simulink model "clik_inverse"  (R2024b)
settings: Solver=ode1  StartTime=0.0  StopTime=4  FixedStep=0.001  RelTol=1e-3
undefined symbols (not defined in the file or in its folder): DiscIntNeverNeededParam, q0, Tc
settings Model: Creator=Xp  LastModifiedBy=22guo
settings SolverCC: AlgebraicLoopSolver=TrustRegion
settings DataIOCC: LimitDataPoints=on  SaveFormat=Array  SignalLoggingSaveFormat=ModelDataLogs  ReturnWorkspaceOutputs=off
settings OptimizationCC: ExpressionDepthLimit=2147483647  InitFltsAndDblsToZero=on  LifeSpan=inf
settings DebuggingCC: SaveWithParameterizedLinksMsg=none  UnderspecifiedInitializationDetection=Classic  MergeDetectMultiDrivingBlocksExec=none  SolverPrmCheckMsg=warning  MultiTaskDSMMsg=warning  MultiTaskCondExecSysMsg=none  FcnCallInpInsideContextMsg=warning  UnconnectedInputMsg=warning  UnconnectedOutputMsg=warning  UnconnectedLineMsg=warning  StateNameClashWarn=warning  SFUnexpectedBacktrackingDiag=warning  SFNoUnconditionalDefaultTransitionDiag=warning  SFExecutionAtInitializationDiag=none  ArithmeticOperatorsInVariantConditions=warning
settings HardwareCC: ProdBitPerPointer=32  ProdBitPerSizeT=32  ProdBitPerPtrDiffT=32  ProdLargestAtomicFloat=None  ProdIntDivRoundTo=Undefined  ProdEndianess=Unspecified  ProdWordSize=32  ProdHWDeviceType=32-bit Generic
settings ModelReferenceCC: EnableRefExpFcnMdlSchedulingChecks=on  PropagateSignalLabelsOutOfModel=off
settings SFSimCC: CustomCodeUndefinedFunction=UseInterfaceOnly
settings RTWCC: GPUComputeCapability=3.5  DLArmComputeVersion=19.05
settings CodeAppCC: StateflowObjectComments=on
settings GRTTargetCC: TargetLangStandard=C89/C90 (ANSI)  CombineOutputUpdateFcns=off  GRTInterface=on
settings ConfigComp: CovMetricSettings=dw  CovSaveCumulativeToWorkspaceVar=on  CovSaveSingleToWorkspaceVar=on

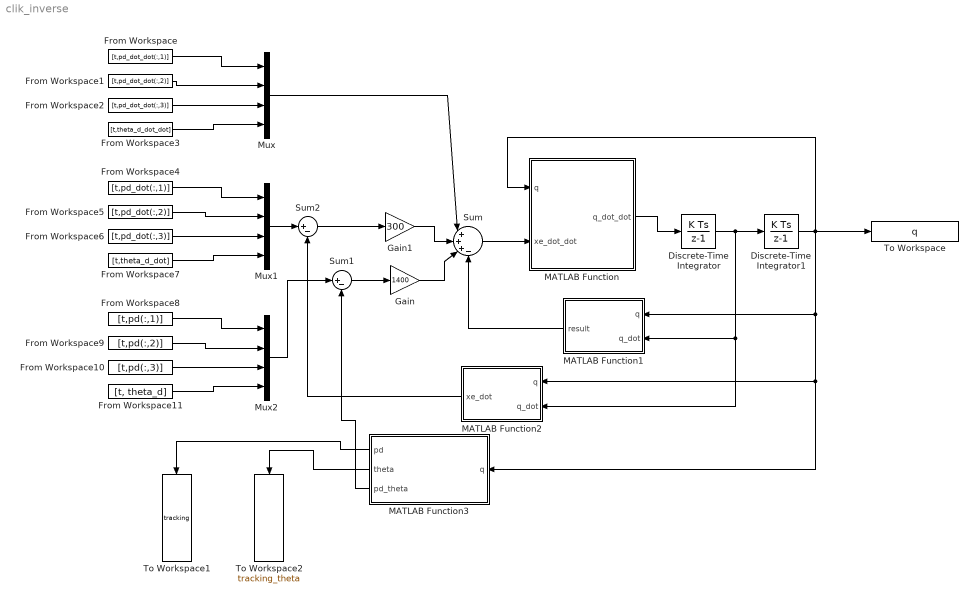
== system clik_inverse ==
  Discrete-Time Integrator : DiscreteIntegrator  SampleTime=Tc  ICPrevOutput=DiscIntNeverNeededParam  ICPrevScaledInput=DiscIntNeverNeededParam
  Discrete-Time Integrator1 : DiscreteIntegrator  InitialCondition=q0  SampleTime=-1  ICPrevOutput=DiscIntNeverNeededParam  ICPrevScaledInput=DiscIntNeverNeededParam
  From Workspace : FromWorkspace  VariableName=[t,pd_dot_dot(:,1)]  SampleTime=Tc
  From Workspace1 : FromWorkspace  VariableName=[t,pd_dot_dot(:,2)]  SampleTime=Tc
  From Workspace10 : FromWorkspace  VariableName=[t,pd(:,3)]  SampleTime=0.001
  From Workspace11 : FromWorkspace  VariableName=[t, theta_d]  SampleTime=0.001
  From Workspace2 : FromWorkspace  VariableName=[t,pd_dot_dot(:,3)]  SampleTime=Tc
  From Workspace3 : FromWorkspace  VariableName=[t,theta_d_dot_dot]  SampleTime=Tc
  From Workspace4 : FromWorkspace  VariableName=[t,pd_dot(:,1)]  SampleTime=Tc
  From Workspace5 : FromWorkspace  VariableName=[t,pd_dot(:,2)]  SampleTime=Tc
  From Workspace6 : FromWorkspace  VariableName=[t,pd_dot(:,3)]  SampleTime=Tc
  From Workspace7 : FromWorkspace  VariableName=[t,theta_d_dot]  SampleTime=Tc
  From Workspace8 : FromWorkspace  VariableName=[t,pd(:,1)]  SampleTime=0.001
  From Workspace9 : FromWorkspace  VariableName=[t,pd(:,2)]  SampleTime=0.001
  Gain : Gain  Gain=1400
  Gain1 : Gain  Gain=300
  MATLAB Function : MATLAB Function  TreatAsAtomicUnit=on
  MATLAB Function1 : MATLAB Function  TreatAsAtomicUnit=on
  MATLAB Function2 : MATLAB Function  TreatAsAtomicUnit=on
  MATLAB Function3 : MATLAB Function  TreatAsAtomicUnit=on
  Mux : Mux
  Mux1 : Mux
  Mux2 : Mux
  Sum : Sum  Inputs=|+++-
  Sum1 : Sum  Inputs=|+-
  Sum2 : Sum  Inputs=|+-
  To Workspace : ToWorkspace  VariableName=q  SampleTime=-1
  To Workspace1 : ToWorkspace  VariableName=tracking  SampleTime=-1
      settings: Save2DSignal=2-D array (concatenate along first dimension)
  To Workspace2 : ToWorkspace  VariableName=tracking_theta  SampleTime=-1
      settings: Save2DSignal=2-D array (concatenate along first dimension)
  wires:
  Discrete-Time Integrator/1 -> MATLAB Function1/2(q_dot), MATLAB Function2/2(q_dot), Discrete-Time Integrator1/1
  From Workspace/1 -> Mux/1
  From Workspace1/1 -> Mux/2
  From Workspace2/1 -> Mux/3
  From Workspace3/1 -> Mux/4
  From Workspace4/1 -> Mux1/1
  From Workspace6/1 -> Mux1/3
  From Workspace5/1 -> Mux1/2
  From Workspace7/1 -> Mux1/4
  From Workspace8/1 -> Mux2/1
  From Workspace10/1 -> Mux2/3
  From Workspace9/1 -> Mux2/2
  From Workspace11/1 -> Mux2/4
  Mux1/1 -> Sum2/1
  Sum2/1 -> Gain1/1
  MATLAB Function2/1(xe_dot) -> Sum2/2
  Gain1/1 -> Sum/2
  Mux/1 -> Sum/1
  Sum1/1 -> Gain/1
  Mux2/1 -> Sum1/1
  Gain/1 -> Sum/3
  MATLAB Function1/1(result) -> Sum/4
  Sum/1 -> MATLAB Function/2(xe_dot_dot)
  MATLAB Function/1(q_dot_dot) -> Discrete-Time Integrator/1
  Discrete-Time Integrator1/1 -> MATLAB Function3/1(q), MATLAB Function2/1(q), MATLAB Function1/1(q), To Workspace/1, MATLAB Function/1(q)
  MATLAB Function3/3(pd_theta) -> Sum1/2
  MATLAB Function3/2(theta) -> To Workspace2/1
  MATLAB Function3/1(pd) -> To Workspace1/1

== matlab function clik_inverse/MATLAB Function ==
  data: q input; xe_dot_dot input; q_dot_dot output
function q_dot_dot = J_inverse(q,xe_dot_dot)
q_dot_dot = jacobian_inverse (q, xe_dot_dot);
end

== matlab function clik_inverse/MATLAB Function2 ==
  data: q input; xe_dot output; q_dot input
function xe_dot = J(q,q_dot)

    a1 = 0.5; 
    a2 = 0.5;

    % extract joints from q
    theta1 = q(1);  
    theta2 = q(2);  

  J = [
        -a1 * sin(theta1) - a2 * sin(theta1 + theta2), -a2 * sin(theta1 + theta2), 0, 0;
         a1 * cos(theta1) + a2 * cos(theta1 + theta2),  a2 * cos(theta1 + theta2), 0, 0;
         0, 0, -1, 0;
         1, 1 0, 1
    ];


  xe_dot=J*q_dot;


end

== matlab function clik_inverse/MATLAB Function3 ==
  data: q input; pd output; theta output; pd_theta output
function [pd,theta,pd_theta] = direct_kin(q)
[pd, theta, pd_theta]= direct_kin(q);
end

== matlab function clik_inverse/MATLAB Function1 ==
  data: q input; result output; q_dot input
function result = J_dot(q,q_dot)
 result = jacobian_dot(q,q_dot);
end
